simulink model "district_model"  (R2026a)
settings: Solver=VariableStepAuto  StopTime=districtSimulationDurationDays * 86400
undefined symbols (not defined in the file or in its folder): coder, districtSimulationLog, m, n, timeStamp
settings Model: Creator=jitheswar  LastModifiedBy=jitheswar

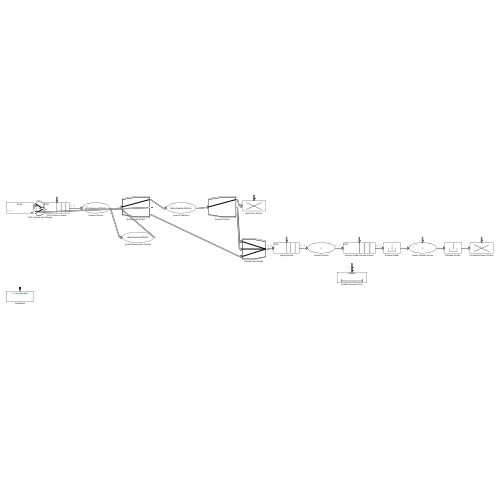
[thumbnail: Simulink's stored preview of the top-level diagram]
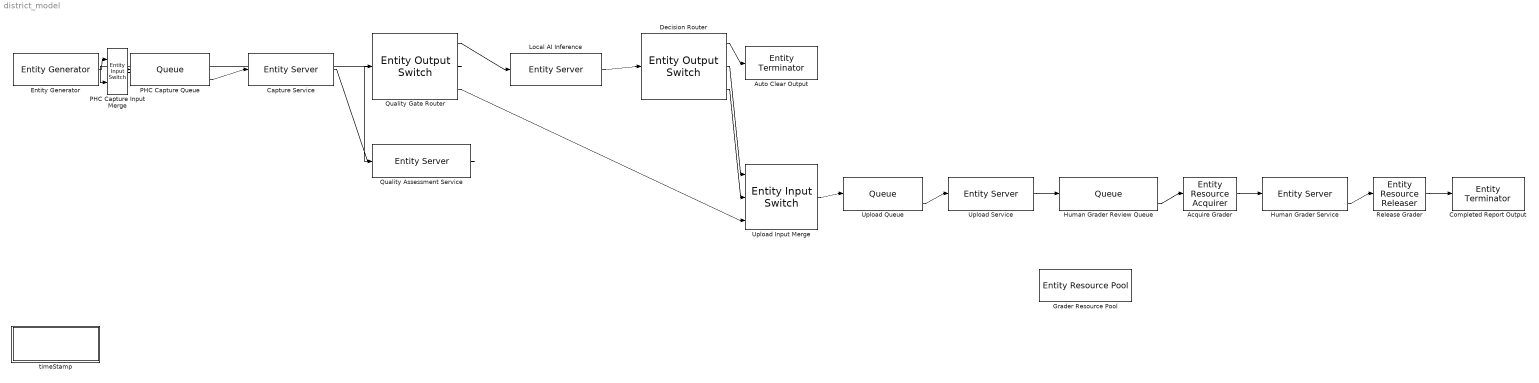
== system district_model ==
  Acquire Grader : EntityResourceAcquirer  InputPortMessageModes=m  OutputPortMessageModes=m  ResourceName=Graders
      settings: OutputPortMap=o3
  Auto Clear Output : EntityTerminator  InputPortMessageModes=m  NumberEntitiesArrived=on
      settings: OutputPortMap=o0
  Capture Service : EntityServer  InputPortMessageModes=m  OutputPortMessageModes=m  Capacity=districtNumberOfPHCs  ServiceTimeValue=districtCaptureTimeSeconds  ServiceCompleteAction=coder.extrinsic('districtSimulationLog', 'rand'); entity.AttemptNumber = entity.AttemptNumber + 1; qualityDraw = 0; qualityDraw = rand(1,1); if districtQualityGateEnabled, entity.QualityFailed = double(qualityDraw < districtQualityRejectionRate); else, entity.QualityFailed = 0; end; if entity.QualityFailed && entity.AttemptNumber <= districtMaximumRecaptureAttempts, entity.QualityRoute = 2; elseif entity.QualityFailed, entity.QualityRoute = 3; else, entity.QualityRoute = 1; end; districtSimulationLog('quality', entity.QualityFailed, entity.AttemptNumber, districtMaximumRecaptureAttempts);
  Completed Report Output : EntityTerminator  InputPortMessageModes=m  NumberEntitiesArrived=on
      settings: OutputPortMap=o0
  Decision Router : EntityOutputSwitch  InputPortMessageModes=m  OutputPortMessageModes=m,m,m  NumberOutputPorts=3  SwitchingCriterion=From attribute  SwitchAttributeName=DecisionRoute
      settings: OutputPortMap=o0,o1,o2
  Entity Generator : EntityGenerator  OutputPortMessageModes=m  TimeSource=MATLAB action  IntergenerationTimeAction=coder.extrinsic('districtNextArrival'); dt = 0; dt = double(districtNextArrival(districtArrivalRate, districtArrivalModeCode, districtCampBurstMultiplier));  GenerateEntityAtSimulationStart=off  GenerateAction=coder.extrinsic('districtSimulationLog'); entity.ArrivalTime = timeStamp(); districtSimulationLog('generated'); entity.AttemptNumber = 0; entity.QualityRoute = 1; entity.DecisionRoute = 1;  AttributeName=PatientID|ArrivalTime|AttemptNumber|QualityFailed|QualityRoute|DecisionRoute  AttributeInitialValue=0|0|0|0|1|1  EntityType=Structured  EntityTypeName=Entity
  Grader Resource Pool : EntityResourcePool  ResourceName=Graders  ResourceAmount=districtNumberOfGraders  AmountInUse=on  AverageUtilization=on
      settings: OutputPortMap=o0,o1
  Human Grader Review Queue : Queue  InputPortMessageModes=m  OutputPortMessageModes=n,m  Capacity=inf  EntryAction=coder.extrinsic('districtSimulationLog'); districtSimulationLog('queue', 3, 1, timeStamp());  ExitAction=coder.extrinsic('districtSimulationLog'); districtSimulationLog('queue', 3, -1, timeStamp());  NumberEntitiesInBlock=on
      settings: OutputPortMap=o1,o5
  Human Grader Service : EntityServer  InputPortMessageModes=m  OutputPortMessageModes=n,m  Capacity=1  ServiceTimeValue=districtGraderServiceTimeSeconds  ServiceCompleteAction=coder.extrinsic('districtSimulationLog'); now = timeStamp(); districtSimulationLog('completed', now - entity.ArrivalTime, districtGraderServiceTimeSeconds);  Utilization=on
      settings: OutputPortMap=o5,o9
  Local AI Inference : EntityServer  InputPortMessageModes=m  OutputPortMessageModes=m  Capacity=districtNumberOfPHCs  ServiceTimeValue=districtInferenceTimeSeconds  ServiceCompleteAction=coder.extrinsic('districtSimulationLog', 'rand'); deferralDraw = 0; deferralDraw = rand(1,1); prevalenceDraw = 0; prevalenceDraw = rand(1,1); operatingDraw = 0; operatingDraw = rand(1,1); if deferralDraw < districtDeferralRate, entity.DecisionRoute = 3; else, hasDisease = prevalenceDraw < districtReferablePrevalence; if hasDisease && operatingDraw < districtModelSensitivity, entity.DecisionRoute = 2; elseif ~hasDisease && operatingDraw > districtModelSpecificity, entity.DecisionRoute = 2; else, entity.DecisionRoute = 1; end; end; districtSimulationLog('decision', entity.DecisionRoute);
  PHC Capture Input Merge : EntityInputSwitch  InputPortMessageModes=m,m  OutputPortMessageModes=m
  PHC Capture Queue : Queue  InputPortMessageModes=m  OutputPortMessageModes=n,m  Capacity=inf  EntryAction=coder.extrinsic('districtSimulationLog'); districtSimulationLog('queue', 1, 1, timeStamp());  ExitAction=coder.extrinsic('districtSimulationLog'); districtSimulationLog('queue', 1, -1, timeStamp());  NumberEntitiesInBlock=on
      settings: OutputPortMap=o1,o5
  Quality Assessment Service : EntityServer  InputPortMessageModes=m  OutputPortMessageModes=m  Capacity=districtNumberOfPHCs  ServiceTimeValue=districtQualityGateTimeSeconds
  Quality Gate Router : EntityOutputSwitch  InputPortMessageModes=m  OutputPortMessageModes=m,m,m  NumberOutputPorts=3  SwitchingCriterion=From attribute  SwitchAttributeName=QualityRoute
      settings: OutputPortMap=o0,o1,o2
  Release Grader : EntityResourceReleaser  InputPortMessageModes=m  OutputPortMessageModes=m
  Upload Input Merge : EntityInputSwitch  InputPortMessageModes=m,m,m  OutputPortMessageModes=m  NumberInputPorts=3
      settings: InputPortMap=u1,u2,u3
  Upload Queue : Queue  InputPortMessageModes=m  OutputPortMessageModes=n,m  Capacity=inf  EntryAction=coder.extrinsic('districtSimulationLog'); districtSimulationLog('queue', 2, 1, timeStamp());  ExitAction=coder.extrinsic('districtSimulationLog'); districtSimulationLog('queue', 2, -1, timeStamp());  NumberEntitiesInBlock=on
      settings: OutputPortMap=o1,o5
  Upload Service : EntityServer  InputPortMessageModes=m  OutputPortMessageModes=m  Capacity=1  ServiceTimeSource=MATLAB action  ServiceTimeAction=tx = districtImageSizeMegabytes * 8 / districtBandwidthMegabitsPerSecond; cycle = districtConnectivityCycleSeconds; phase = mod(timeStamp(), cycle); window = districtConnectivityAvailability * cycle; if phase < window, dt = tx; else, dt = (cycle - phase) + tx; end;
  timeStamp : Subsystem  TreatAsAtomicUnit=on
  wires:
  Entity Generator/1 -> PHC Capture Input Merge/1
  PHC Capture Input Merge/1 -> PHC Capture Queue/1
  PHC Capture Queue/2 -> Capture Service/1
  Capture Service/1 -> Quality Assessment Service/1
  Quality Assessment Service/1 -> Quality Gate Router/1
  Quality Gate Router/1 -> Local AI Inference/1
  Quality Gate Router/2 -> PHC Capture Input Merge/2
  Quality Gate Router/3 -> Upload Input Merge/3
  Local AI Inference/1 -> Decision Router/1
  Decision Router/1 -> Auto Clear Output/1
  Decision Router/2 -> Upload Input Merge/1
  Decision Router/3 -> Upload Input Merge/2
  Upload Input Merge/1 -> Upload Queue/1
  Upload Queue/2 -> Upload Service/1
  Upload Service/1 -> Human Grader Review Queue/1
  Human Grader Review Queue/2 -> Acquire Grader/1
  Acquire Grader/1 -> Human Grader Service/1
  Human Grader Service/2 -> Release Grader/1
  Release Grader/1 -> Completed Report Output/1

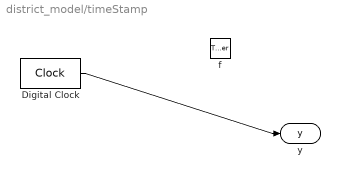
== system district_model/timeStamp ==
  f : TriggerPort  TriggerType=function-call  IsSimulinkFunction=on  FunctionName=timeStamp  FunctionVisibility=scoped  VariantControl=(inherit)
  Digital Clock : DigitalClock  SampleTime=-1
  y : ArgOut  DisableCoverage=on  ArgumentName=y
  wires:
  Digital Clock/1 -> y/1
